simulink model "eg2"  (R2015a)
settings: Solver=ode45  StartTime=0.0  StopTime=100  RelTol=1e-3
libraries: simulink x1
settings Model: Creator=ayush  LastModifiedBy=ayush

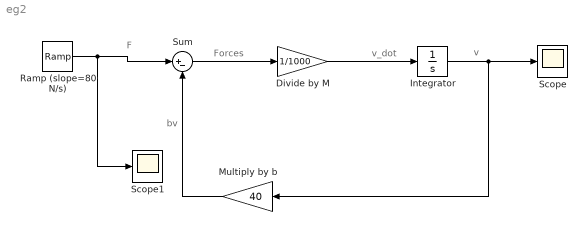
== system eg2 ==
  note: bv
  note: v
  note: v_dot
  note: Forces
  note: F
  Divide by M : Gain  Gain=1/1000
  Integrator : Integrator
  Multiply by b : Gain  Gain=40
  Ramp (slope=80 N/s) : simulink/Sources/Ramp  slope=80  start=0  X0=0
  Scope : Scope
  Scope1 : Scope
  Sum : Sum  Inputs=|+-
  wires:
  Sum/1 -> Divide by M/1
  Divide by M/1 -> Integrator/1
  Integrator/1 -> Multiply by b/1, Scope/1
  Multiply by b/1 -> Sum/2
  Ramp (slope=80 N/s)/1 -> Scope1/1, Sum/1
